simulink model "Proyecto_Simulacion"  (R2023a)
settings: Solver=VariableStepAuto  StartTime=0.0  StopTime=1000  RelTol=1e-3
undefined symbols (not defined in the file or in its folder): m, n
settings Model: Creator=mluser

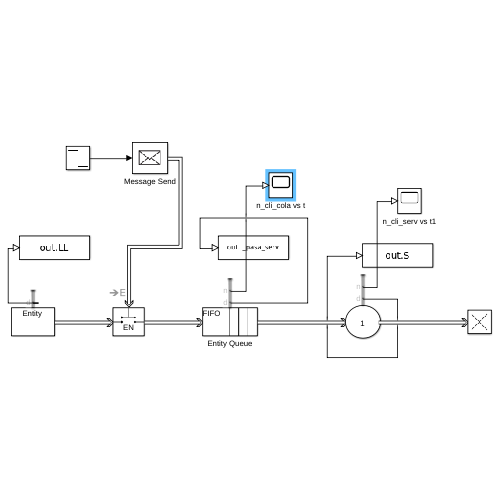
[thumbnail: Simulink's stored preview of the top-level diagram]
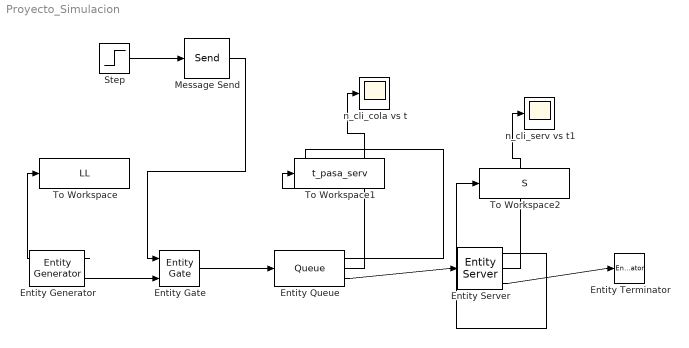
== system Proyecto_Simulacion ==
  Entity Gate : EntityGate  InputPortMessageModes=m,m  OutputPortMessageModes=m
  Entity Generator : EntityGenerator  OutputPortMessageModes=n,m  TimeSource=MATLAB action  IntergenerationTimeAction=|  NumberEntitiesDeparted=on  EntityType=Structured  EntityTypeName=Entity
      | value = 1
      | value = rand()
      | mu = 2
      | dt = -mu*log(1-value)
      settings: OutputPortMap=o0,o3
  Entity Queue : Queue  InputPortMessageModes=m  OutputPortMessageModes=n,n,m  Capacity=inf  NumberEntitiesDeparted=on  NumberEntitiesInBlock=on
      settings: OutputPortMap=o0,o1,o5
  Entity Server : EntityServer  InputPortMessageModes=m  OutputPortMessageModes=n,n,m  Capacity=1  ServiceTimeSource=MATLAB action  ServiceTimeAction=|  NumberEntitiesDeparted=on  NumberEntitiesInBlock=on
      | value = 1
      | value = rand()
      | mu = 3
      | dt = -mu*log(1-value)
      settings: OutputPortMap=o0,o1,o9
  Entity Terminator : EntityTerminator  InputPortMessageModes=m
  Message Send : Send  OutputPortMessageModes=m
  Step : Step  Time=180  Before=1  After=0  SampleTime=0
  To Workspace : ToWorkspace  VariableName=LL  SaveFormat=Timeseries  SampleTime=-1
  To Workspace1 : ToWorkspace  VariableName=t_pasa_serv  SaveFormat=Timeseries  SampleTime=-1
  To Workspace2 : ToWorkspace  VariableName=S  SaveFormat=Timeseries  SampleTime=-1
  n_cli_cola vs t : Scope
  n_cli_serv vs t1 : Scope
  wires:
  Step/1 -> Message Send/1
  Message Send/1 -> Entity Gate/1
  Entity Generator/2 -> Entity Gate/2
  Entity Gate/1 -> Entity Queue/1
  Entity Generator/1 -> To Workspace/1
  Entity Queue/3 -> Entity Server/1
  Entity Server/3 -> Entity Terminator/1
  Entity Server/1 -> To Workspace2/1
  Entity Queue/1 -> To Workspace1/1
  Entity Queue/2 -> n_cli_cola vs t/1
  Entity Server/2 -> n_cli_serv vs t1/1
